simulink library "surfaceCoefficients_ul"  (R2018b)
settings: Solver=VariableStepAuto  StartTime=0.0  StopTime=10.0  RelTol=1e-3
libraries: dsppolyfun x2
settings Model: Creator=mcobb  LastModifiedBy=asiddiq2

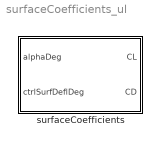
== system surfaceCoefficients_ul ==
  surfaceCoefficients : Subsystem  mask{CLvals=[-1 0 1]', CDvals=[02 0.1 0.2]', alphaVals=[-10 0 10]', GainCL=[0 0.1 0], GainCD=[0 0.01 0]}
      mask prompts: CLvals "CL values"; CDvals "CD values"; alphaVals "Angle of attack values"; GainCL "Control surface CL gain"; GainCD "Control surface CD gain"

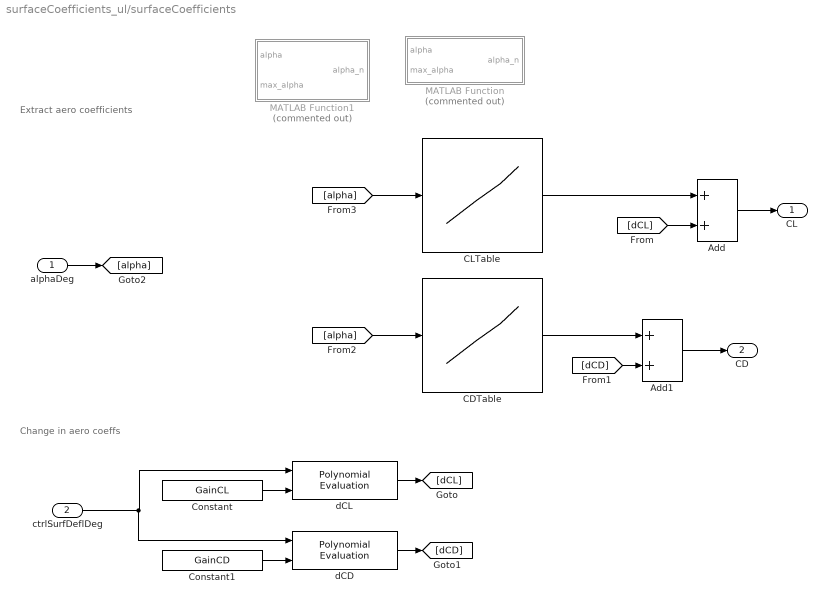
== system surfaceCoefficients_ul/surfaceCoefficients ==
  note: Change in aero coeffs
  note: Extract aero coefficients
  alphaDeg : Inport
  ctrlSurfDeflDeg : Inport  Port=2
  Add : Sum
  Add1 : Sum
  CDTable : Lookup_n-D  NumberOfTableDimensions=1  LookupTableObject=CLTable  BreakpointsForDimension1=alphaVals  Table=CDvals  ExtrapMethod=Clip  UseLastTableValue=on  InternalRulePriority=Speed  RndMeth=Simplest  InputSameDT=on
  CLTable : Lookup_n-D  NumberOfTableDimensions=1  LookupTableObject=CLTable  BreakpointsForDimension1=alphaVals  Table=CLvals  ExtrapMethod=Clip  UseLastTableValue=on  InternalRulePriority=Speed  RndMeth=Simplest  InputSameDT=on
  Constant : Constant  Value=GainCL  VectorParams1D=off
  Constant1 : Constant  Value=GainCD  VectorParams1D=off
  MATLAB Function : MATLAB Function  Commented=on  TreatAsAtomicUnit=on
  MATLAB Function1 : MATLAB Function  Commented=on  TreatAsAtomicUnit=on
  dCD : dsppolyfun/Polynomial Evaluation  useConstCoeffs=off  constCoeffs=[0]
      settings: SourceProductName=DSP System Toolbox  SourceProductBaseCode=DS
  dCL : dsppolyfun/Polynomial Evaluation  useConstCoeffs=off  constCoeffs=[0]
      settings: SourceProductName=DSP System Toolbox  SourceProductBaseCode=DS
  CL : Outport
  CD : Outport  Port=2
  wires:
  alphaDeg/1 -> [alpha]
  dCL/1 -> [dCL]
  dCD/1 -> [dCD]
  [dCL] -> Add/2
  Add/1 -> CL/1
  Add1/1 -> CD/1
  [dCD] -> Add1/2
  CDTable/1 -> Add1/1
  Constant/1 -> dCL/2
  Constant1/1 -> dCD/2
  ctrlSurfDeflDeg/1 -> dCD/1, dCL/1
  [alpha] -> CDTable/1
  CLTable/1 -> Add/1
  [alpha] -> CLTable/1

== matlab function surfaceCoefficients_ul/surfaceCoefficients/MATLAB Function1 ==
  data: alpha input; alpha_n output; max_alpha input
function alpha_n = fcn(alpha,max_alpha)

if abs(alpha)>=max_alpha
    alpha_n = max_alpha;
else
    alpha_n = alpha;
end
end

== matlab function surfaceCoefficients_ul/surfaceCoefficients/MATLAB Function ==
  data: alpha input; alpha_n output; max_alpha input
function alpha_n = fcn(alpha,max_alpha)

if abs(alpha)>=max_alpha
    alpha_n = 0;
else
    alpha_n = alpha;
end
end
